simulink model "doc_softdecision"  (Simulink 4.00)
settings: Solver=ode45  SolverMode=SingleTasking  StartTime=0.0  StopTime=inf  RelTol=1e-3
undefined symbols (not defined in the file): slcm
libraries: commcnvcod2 x2, commchan2 x1, commdigbbndpm2 x1, commsource2 x1, commsink2 x1, dspstat3 x1, dspquant2 x1
settings Model: RequirementInfo=9  CovMetricSettings=d  Creator=mikem  LastModifiedBy=agaltman  SaveTime=off  SaveOutput=off  SaveFormat=Structure  LimitDataPoints=off  IntegerOverflowMsg=none  TryForceingSFcnDF=off  ExtModeTrigMode=oneshot  ExtModeArmWhenConnect=off  BlockReductionOpt=off

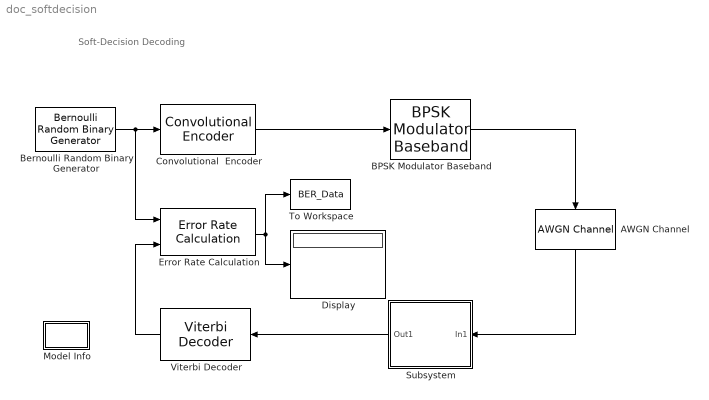
== system doc_softdecision ==
  note: Soft-Decision Decoding
  AWGN Channel : commchan2/AWGN Channel  Orientation=down  seed=1237  noiseMode="Signal to noise ratio  (Es/No)"  EsNodB=-1  SNRdB=10  Ps=1  Tsym=.5  variance=1
  BPSK Modulator Baseband : commdigbbndpm2/BPSK Modulator Baseband  Ph=0  numSamp=1
  Bernoulli Random Binary Generator : commsource2/Bernoulli Random Binary Generator  P=0.5  seed=25741  Ts=1  frameBased=on  sampPerFrame=10000  orient=off
  Convolutional  Encoder : commcnvcod2/Convolutional Encoder  trellis=poly2trellis(7, [171 133])  reset=None
  Display : Display
      settings: Format=short
  Error Rate Calculation : commsink2/Error Rate Calculation  N=48  st_delay=0  cp_mode=Entire frame  subframe=[]  PMode=Port  WsName=ErrorVec  RsMode2=off  stop=on  numErr=100  maxBits=1e7
  Model Info : Subsystem  LoadFcn=slcm LoadBlock;  InitFcn=slcm('UpdateAllCMBlocksInThisModelInit')  mask(CMBlock){InitialSaveTempField=, InitialBlockCM=none, BlockCM=none, Frame=on, SaveTempField=, DisplayStringWithTags=Info, MaskDisplayString=Info, HorizontalTextAlignment=Center, LeftAlignmentValue=0.5, SourceBlockDiagram=doc_softdecision, TagMaxNumber=20, CMTag1=, CMTag2=, CMTag3=, CMTag4=, CMTag5=, CMTag6=, CMTag7=, CMTag8=, CMTag9=, CMTag10=, CMTag11=, CMTag12=, CMTag13=, CMTag14=, CMTag15=, CMTag16=, CMTag17=, CMTag18=, CMTag19=, CMTag20=}
      mask help: This block allows revision control information to be displayed within the model.
      settings: CopyFcn=slcm CopyBlock;  DeleteFcn=slcm Cancel;  PostSaveFcn=slcm('UpdateAllCMBlocksInThisModel')  NameChangeFcn=slcm Rename;  OpenFcn=commdemohelp;  RTWFcnNameOpts=Auto  RTWFileNameOpts=Auto
      mask Display: text(str2num(LeftAlignmentValue), 0.5, MaskDisplayString, 'HorizontalAlignment', HorizontalTextAlignment)
  Subsystem : Subsystem  Orientation=left
      settings: RTWFcnNameOpts=Auto  RTWFileNameOpts=Auto
      mask Display: disp('Soft-Output\nBPSK\nDemodulator')
  To Workspace : ToWorkspace  VariableName=BER_Data  SampleTime=-1  SaveFormat=Array
      settings: MaxDataPoints=1
  Viterbi Decoder : commcnvcod2/Viterbi Decoder  Orientation=left  trellis=poly2trellis(7, [171 133])  dectype=Soft Decision  nsdecb=3  tbdepth=48  opmode=Continuous  reset=off
  wires:
  Convolutional  Encoder/1 -> BPSK Modulator Baseband/1
  BPSK Modulator Baseband/1 -> AWGN Channel/1
  Bernoulli Random Binary Generator/1 -> Convolutional  Encoder/1, Error Rate Calculation/1
  Error Rate Calculation/1 -> Display/1, To Workspace/1
  Viterbi Decoder/1 -> Error Rate Calculation/2
  AWGN Channel/1 -> Subsystem/1(In1)
  Subsystem/1(Out1) -> Viterbi Decoder/1

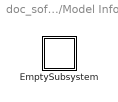
== system doc_softdecision/Model Info ==
  EmptySubsystem : Subsystem
      settings: RTWFcnNameOpts=Auto  RTWFileNameOpts=Auto

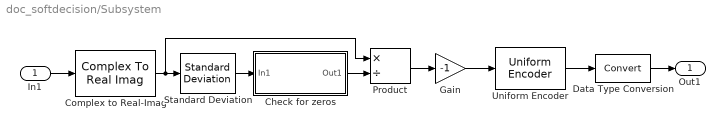
== system doc_softdecision/Subsystem ==
  In1 : Inport  Port=1
  Check for zeros : Subsystem
      settings: RTWFcnNameOpts=Auto  RTWFileNameOpts=Auto
      mask Display: disp('Check for zeros')
  Complex to Real-Imag : ComplexToRealImag  Output=Real
  Data Type Conversion : DataTypeConversion  DataType=auto  SaturateOnIntegerOverflow=on
  Gain : Gain  Gain=-1  Multiplication=Element-wise(K.*u)  SaturateOnIntegerOverflow=on
  Product : Product  Inputs=*/  Multiplication=Element-wise(.*)  SaturateOnIntegerOverflow=on
  Standard Deviation : dspstat3/Standard Deviation  run=on  reset_popup=None
  Uniform Encoder : dspquant2/Uniform Encoder  peak=2  bits=3  otype=Unsigned integer
  Out1 : Outport  Port=1
  wires:
  Check for zeros/1(Out1) -> Product/2
  In1/1 -> Complex to Real-Imag/1
  Standard Deviation/1 -> Check for zeros/1(In1)
  Complex to Real-Imag/1 -> Standard Deviation/1, Product/1
  Uniform Encoder/1 -> Data Type Conversion/1
  Gain/1 -> Uniform Encoder/1
  Product/1 -> Gain/1
  Data Type Conversion/1 -> Out1/1

== system doc_softdecision/Model Info/EmptySubsystem ==

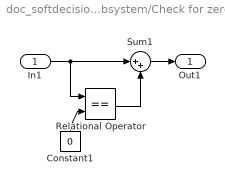
== system doc_softdecision/Subsystem/Check for zeros ==
  In1 : Inport  Port=1
  Constant1 : Constant  Orientation=up  Value=0
  Relational Operator : RelationalOperator  Operator===
  Sum1 : Sum  Inputs=|++  SaturateOnIntegerOverflow=on
  Out1 : Outport  Port=1
  wires:
  Relational Operator/1 -> Sum1/2
  Constant1/1 -> Relational Operator/2
  Sum1/1 -> Out1/1
  In1/1 -> Relational Operator/1, Sum1/1
